simulink model "model"  (R2024a)
settings: Solver=VariableStepAuto  StartTime=0.0  StopTime=5  RelTol=1e-3
values from neighbouring files (symbols this model uses):
  k = 0.5    [design_mpc.m]
  m = 10    [design_mpc.m]
  Ts = 0.1    [design_mpc.m]
libraries: simulink x1, mpclib x1
settings Model: Creator=berto  LastModifiedBy=berto

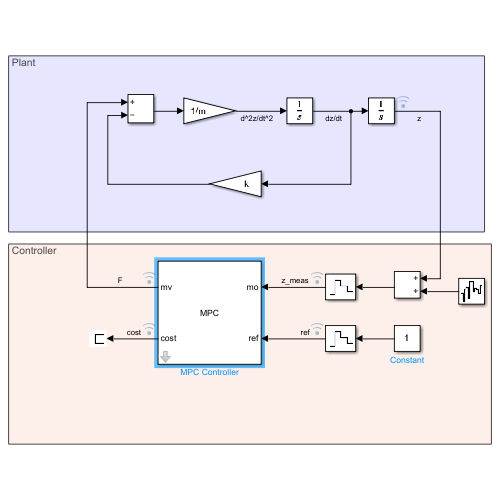
[thumbnail: Simulink's stored preview of the top-level diagram]
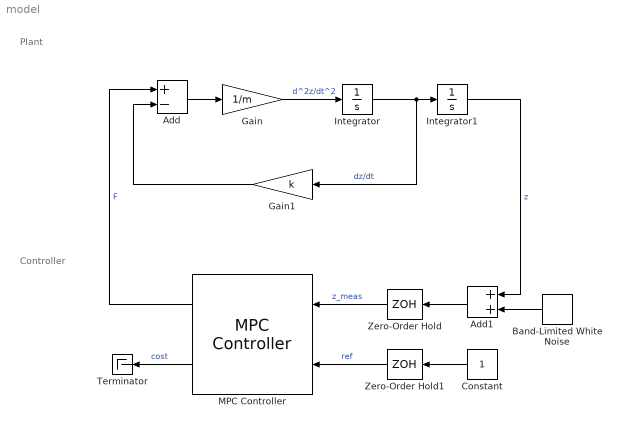
== system model ==
  note: Controller
  note: Plant
  Add : Sum  Inputs=+-
  Add1 : Sum
  Band-Limited White Noise : simulink/Sources/Band-Limited White Noise  Cov=[0.0005]  Ts=Ts  seed=[23341]
  Constant : Constant
  Gain : Gain  Gain=1/m
  Gain1 : Gain  Gain=k
  Integrator : Integrator
  Integrator1 : Integrator
  MPC Controller : mpclib/MPC Controller  SCDEnableBlockLinearizationSpecification=on  mpcobj=mpcobj  is_multiple=0  enable_value=0  return_u0=off  updateMPCinCallerWorkspace=on  md_inport=off  mv_inport=off  uref_inport=off  return_cost=on  return_mvseq=off  return_qpstatus=off  return_xseq=off  return_state=off  return_ovseq=off  state_inport=off  umin_inport=off  umax_inport=off  ymin_inport=off  ymax_inport=off  cc_inport=off  ywt_inport=off  uwt_inport=off  duwt_inport=off  rhoeps_inport=off  pm_inport=off  MaximumP=10  HorizonChoice=FixedHorizon  n_ts=0.1  n_p=10  n_mv=1  n_md=0  n_ud=0  n_mo=1  n_uo=0  BlockDataType=double  SampleTimeInherited=off  switch_inport=off
  Terminator : Terminator
  Zero-Order Hold : ZeroOrderHold  SampleTime=Ts
  Zero-Order Hold1 : ZeroOrderHold  SampleTime=Ts
  wires:
  Integrator/1 -> Gain1/1, Integrator1/1  "dz/dt"
  Gain/1 -> Integrator/1  "d^2z/dt^2"
  Add/1 -> Gain/1
  Gain1/1 -> Add/2
  Integrator1/1 -> Add1/1  "z"
  MPC Controller/1 -> Add/1  "F"
  Constant/1 -> Zero-Order Hold1/1
  MPC Controller/2 -> Terminator/1  "cost"
  Band-Limited White Noise/1 -> Add1/2
  Add1/1 -> Zero-Order Hold/1
  Zero-Order Hold/1 -> MPC Controller/1  "z_meas"
  Zero-Order Hold1/1 -> MPC Controller/2  "ref"
